simulink model "project1_IM_switch_circuit"  (R2020b)
settings: Solver=ode23tb  StartTime=0.0  StopTime=1.0  MaxStep=10e-6  RelTol=1e-4
libraries: powerlib x13, powerlib_meascontrol x1
Description:
  | Copyright 2008-2015 The MathWorks, Inc.
settings Model: ExtModeTrigMode=oneshot  ExtModeArmWhenConnect=off  ExtModeAutoUpdateStatusClock=off  Creator=MathWorks  LastModifiedBy=tmcnama2
settings DataIOCC: ExternalInput=[]  SaveFormat=Array  SignalLoggingSaveFormat=ModelDataLogs  SaveOutput=off  ReturnWorkspaceOutputs=off  TimeSaveName=t  SignalLoggingName=sigsOut
settings OptimizationCC: BlockReduction=off  BooleanDataType=off  ExpressionDepthLimit=2147483647  InitFltsAndDblsToZero=on  EfficientMapNaN2IntZero=off  LifeSpan=inf
settings DebuggingCC: UnderspecifiedInitializationDetection=Classic  MergeDetectMultiDrivingBlocksExec=none  CheckExecutionContextPreStartOutputMsg=on  CheckExecutionContextRuntimeOutputMsg=on  SignalResolutionControl=TryResolveAllWithWarning  MultiTaskDSMMsg=warning  MultiTaskCondExecSysMsg=none  SigSpecEnsureSampleTimeMsg=none  FcnCallInpInsideContextMsg=warning  UnconnectedInputMsg=none  UnconnectedOutputMsg=none  StateNameClashWarn=warning  SFUnexpectedBacktrackingDiag=warning  SFNoUnconditionalDefaultTransitionDiag=warning  ArithmeticOperatorsInVariantConditions=warning
settings HardwareCC: ProdBitPerPointer=32  ProdBitPerSizeT=32  ProdBitPerPtrDiffT=32  ProdLargestAtomicFloat=None  ProdIntDivRoundTo=Undefined  ProdEndianess=Unspecified  ProdWordSize=32  ProdHWDeviceType=32-bit Generic  TargetUnknown=on
settings ModelReferenceCC: PropagateSignalLabelsOutOfModel=off
settings SFSimCC: SimUseLocalCustomCode=off  CustomCodeUndefinedFunction=UseInterfaceOnly
settings RTWCC: RTWUseLocalCustomCode=off
settings CodeAppCC: StateflowObjectComments=on
settings GRTTargetCC: TargetLangStandard=C89/C90 (ANSI)  CombineOutputUpdateFcns=off  GRTInterface=on
settings ConfigComp: CovMetricSettings=dw  CovSaveCumulativeToWorkspaceVar=on  CovSaveSingleToWorkspaceVar=on  CovExternalEMLEnable=off  CovSFcnEnable=off
settings SimscapeCC: SimscapeNormalizeSystem=off

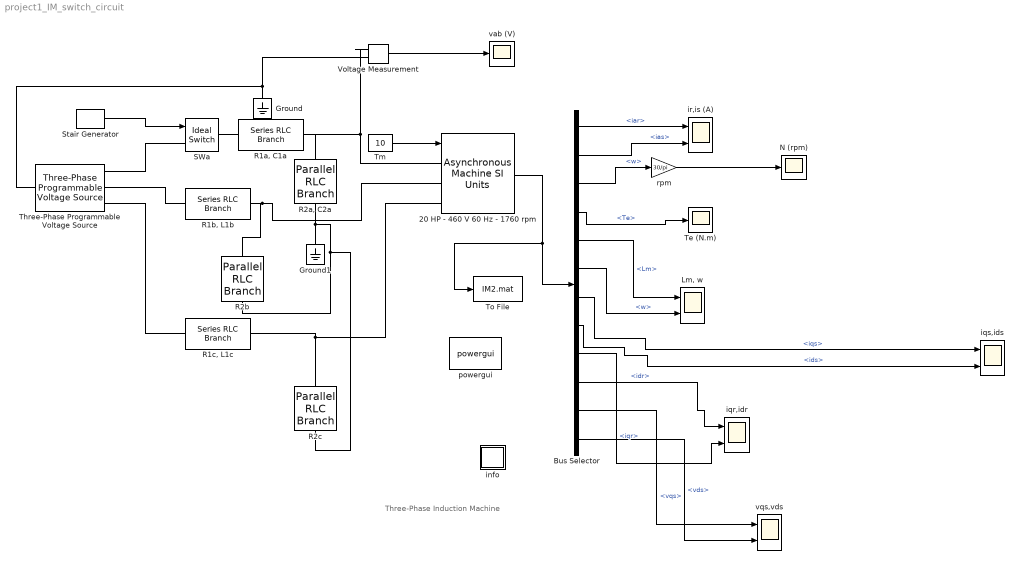
== system project1_IM_switch_circuit ==
  note: Three-Phase Induction Machine
  20 HP - 460 V 60 Hz - 1760 rpm : powerlib/Machines/Asynchronous Machine SI Units  RotorType=Squirrel-cage  PresetModel="03:  20 HP  460 V 60Hz 1760 RPM"  MechanicalLoad=Torque Tm  ShowDetailedParameters=on  ReferenceFrame=Stationary  Units=SI  MeasurementBus=on  NominalParameters=[1.492e+04 460 60]  Stator=[0.2761 0.002191]  Rotor=[0.1645 0.002191]  Cage1=[ 0.022 0.226/377]  Cage2=[ 0.022 0.226/377]  Lm=0.07614  Mechanical=[0.1 0.01771 2]  PolePairs=2  InitialConditions="[ 1,0   0,0,0   0,0,0 ]"  SimulateSaturation=off  Saturation=[14.03593122, 27.81365428, 53.79336849, 72.68890987, 97.98006896, 148.6815601, 215.7428561, 302.9841135, 428.7778367 ; 230, 322, 414, 460, 506, 552, 598, 644, 690]  LoadFlowParameters=0  TsPowergui=0  TsBlock=-1  IterativeModel=Trapezoidal non iterative  IterativeDiscreteModel=Trapezoidal non iterative  Pmec=0
  Bus Selector : BusSelector  OutputSignals=iar,ias,w,Te,Lm,w,iqs,ids,iqr,idr,vqs,vds
  Ground : powerlib/Elements/Ground  LConnTagsString=a
  Ground1 : powerlib/Elements/Ground  LConnTagsString=a
  "Lm, w" : Scope  NumInputPorts=2
  N (rpm) : Scope
  "R1a, C1a" : powerlib/Elements/Series RLC Branch  LConnTagsString=__new0  RConnTagsString=__new0  BranchType=RC  Resistance=0.1  Inductance=10e-6  SetiL0=on  InitialCurrent=0  Capacitance=100e-3  Setx0=off  InitialVoltage=0  Measurements=None
  "R1b, L1b" : powerlib/Elements/Series RLC Branch  LConnTagsString=__new0  RConnTagsString=__new0  BranchType=RL  Resistance=0.1  Inductance=10e-6  SetiL0=on  InitialCurrent=0  Capacitance=1e-6  Setx0=off  InitialVoltage=0  Measurements=None
  "R1c, L1c" : powerlib/Elements/Series RLC Branch  LConnTagsString=__new0  RConnTagsString=__new0  BranchType=RL  Resistance=0.1  Inductance=10e-6  SetiL0=on  InitialCurrent=0  Capacitance=1e-6  Setx0=off  InitialVoltage=0  Measurements=None
  "R2a, C2a" : powerlib/Elements/Parallel RLC Branch  LConnTagsString=a  RConnTagsString=__new0  BranchType=RC  Resistance=100  Inductance=1e-3  SetiL0=off  InitialCurrent=0  Capacitance=100e-6  Setx0=off  InitialVoltage=0  Measurements=None
  R2b : powerlib/Elements/Parallel RLC Branch  LConnTagsString=a  RConnTagsString=__new0  BranchType=R  Resistance=100  Inductance=1e-3  SetiL0=off  InitialCurrent=0  Capacitance=100e-6  Setx0=off  InitialVoltage=0  Measurements=None
  R2c : powerlib/Elements/Parallel RLC Branch  LConnTagsString=a  RConnTagsString=__new0  BranchType=R  Resistance=100  Inductance=1e-3  SetiL0=off  InitialCurrent=0  Capacitance=100e-6  Setx0=off  InitialVoltage=0  Measurements=None
  SWa : powerlib/Power Electronics/Ideal Switch  Ron=0.01  Lon=1e-9  IC=1  Rs=inf  Cs=0  Measurements=off
      settings: AttributesFormatString=\n
  Stair Generator : powerlib_meascontrol/Pulse & Signal Generators/Stair Generator  t="[0 0.7  0.8 ]"  e=[1 0 1]  Ts=0
  Te (N.m) : Scope
  Three-Phase Programmable Voltage Source : powerlib/Electrical Sources/Three-Phase Programmable Voltage Source  PositiveSequence="[460  0 60]"  VariationEntity=None  VariationType=Table of time-amplitude pairs  VariationTypeAlt=Step  VariationStep=0.5  VariationRate=10  VariationMagnitude=0.3  VariationFrequency=2  VariationTiming=[1 2]  VariationPhaseA=off  Amplitudes=[1 0.8 1.2 1.0]  TimeValues=[0 0.1 0.15 0.2]  HarmonicGeneration=off  HarmonicA=[3 0.2 -25 0]  HarmonicB=[2 0.15 35 2]  Timing="[0.05  3]"  BusType=swing  Pref=0  Qref=0  Qmin=-inf  Qmax=inf
  Tm : Constant  Value=10
  To File : ToFile  Filename=IM2.mat  MatrixName=motor_out  SaveFormat=Timeseries
  Voltage Measurement : powerlib/Measurements/Voltage Measurement  PhasorSimulation=off  OutputType=Complex  PSBequivalent=0
  info : Subsystem
      settings: OpenFcn=showdemo(bdroot(gcb))
      mask Display: disp('?')
  iqr,idr : Scope  NumInputPorts=2
  iqs,ids : Scope  NumInputPorts=2
  ir,is (A) : Scope  NumInputPorts=2
  powergui : powerlib/powergui  SimulationMode=Continuous  SampleTime=0  frequency=60  Iterations=50  frequencyindice=60  Pbase=100e6  ErrMax=1e-4  UnitsV=kV  UnitsW=MW  buscounter=0  FunctionMessages=off  echomessages=off  EnableUseOfTLC=off  CurrentSourceSwitches=off  DisableSnubberDevices=off  DisableRonSwitches=off  DisableVfSwitches=off  DisplayEquations=on  AutomaticDiscreteSolvers=off  SolverType=Backward Euler  Interpol=off  ExternalGateDelay=off  methode=off  Ts=0  x0status=blocks  SPID=on  SwTol=0  HookPort=off  NonlinearTolerance=1e-4  nMaxIteration=100  ContinueOnMaxIteration=off  RestoreLinks=warning  ResistiveCurrentMeasurement=off  Frange=[0:2:500]  Ylog=off  Xlog=on  ShowGrid=off  save=off  variable=ZData  structure=0  ZoomFFT=on  StartTime=0.0  cycles=1  DisplayStyle=1  fundamental=60  FreqAxis=off  MaxFrequency=1000  frequencyindicesteady=1  RmsSteady=1  display=off
  rpm : Gain  Gain=30/pi  SaturateOnIntegerOverflow=on  OutDataTypeStr=Inherit: Same as input  ParamDataTypeStr=Inherit: Same as input
  vab (V) : Scope
  vqs,vds : Scope  NumInputPorts=2
  wires:
  Bus Selector/4 -> Te (N.m)/1  "<Te>"
  rpm/1 -> N (rpm)/1
  Tm/1 -> 20 HP - 460 V 60 Hz - 1760 rpm/1
  Bus Selector/1 -> ir,is (A)/1  "<iar>"
  20 HP - 460 V 60 Hz - 1760 rpm/1 -> To File/1, Bus Selector/1
  Bus Selector/2 -> ir,is (A)/2  "<ias>"
  Bus Selector/3 -> rpm/1  "<w>"
  Voltage Measurement/1 -> vab (V)/1
  Bus Selector/5 -> "Lm, w"/1  "<Lm>"
  Bus Selector/6 -> "Lm, w"/2  "<w>"
  Bus Selector/7 -> iqs,ids/1  "<iqs>"
  Bus Selector/8 -> iqs,ids/2  "<ids>"
  Bus Selector/11 -> vqs,vds/1  "<vqs>"
  Bus Selector/12 -> vqs,vds/2  "<vds>"
  Bus Selector/10 -> iqr,idr/1  "<idr>"
  Bus Selector/9 -> iqr,idr/2  "<iqr>"
  Stair Generator/1 -> SWa/1
  connections:
  Voltage Measurement/LConn2 -- Three-Phase Programmable Voltage Source/LConn1 -- Ground/LConn1
  SWa/LConn1 -- Three-Phase Programmable Voltage Source/RConn1
  Voltage Measurement/LConn1 -- "R2a, C2a"/LConn1 -- "R1a, C1a"/RConn1 -- 20 HP - 460 V 60 Hz - 1760 rpm/LConn1
  "R1a, C1a"/LConn1 -- SWa/RConn1
  "R1b, L1b"/LConn1 -- Three-Phase Programmable Voltage Source/RConn2
  "R1b, L1b"/RConn1 -- 20 HP - 460 V 60 Hz - 1760 rpm/LConn2 -- R2b/LConn1
  Three-Phase Programmable Voltage Source/RConn3 -- "R1c, L1c"/LConn1
  "R1c, L1c"/RConn1 -- R2c/LConn1 -- 20 HP - 460 V 60 Hz - 1760 rpm/LConn3
  Ground1/LConn1 -- "R2a, C2a"/RConn1 -- R2c/RConn1 -- R2b/RConn1

== system project1_IM_switch_circuit/info ==
